simulink model "lane_change_acc_model"  (R2023b)
settings: Solver=ode4  StartTime=0.0  StopTime=T  FixedStep=0.1  RelTol=1e-3
InitFcn:
  | dt = 0.1; T = 20;
  | v_ego0 = 15; d_min = 5; t_headway = 1.2;
  | Kp = 0.5;
  | lane_width = 3.5;
  | mode = 1; % mode = 1 (Keep lane), mode = 2 (Change lane)
  | L = 2.8; K_y = 0.2; K_psi = 1.0;
  | del_actual = 0.2; delta_max = 25*pi/180;
  | 
  | % Lead vehicle and ego car's initial conditions
  | x_lead0 = 30; x_ego0 = 0;
  | v_lead0 = 13;
  | y_lead0 = 0; y_ego0 = 0;
libraries: SignalEditorBlockLib x1
settings Model: Creator=HP  LastModifiedBy=HP

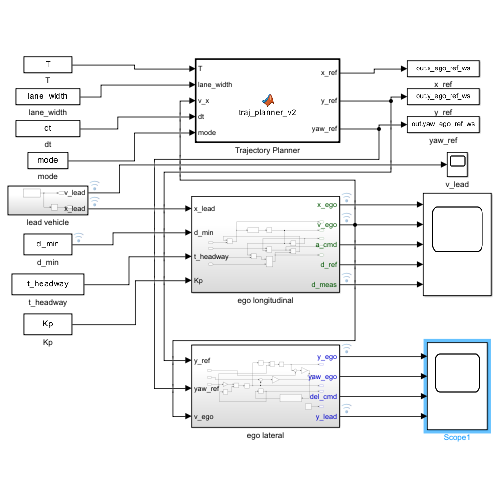
[thumbnail: Simulink's stored preview of the top-level diagram]
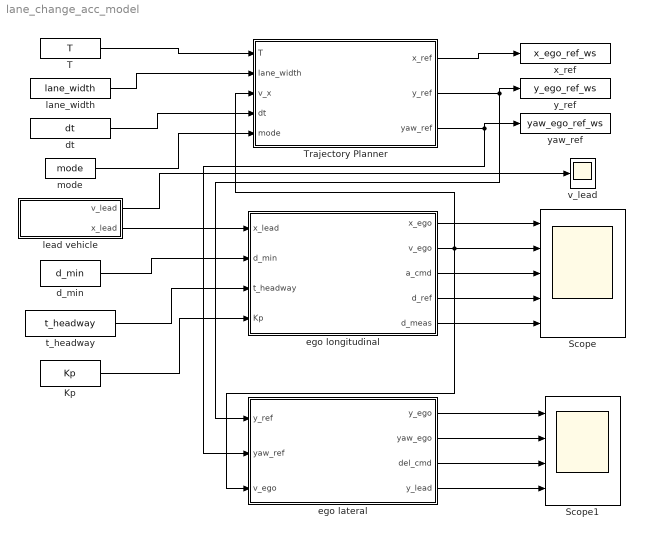
== system lane_change_acc_model ==
  Kp : Constant  Value=Kp
  Scope : Scope  NumInputPorts=5
  Scope1 : Scope  NumInputPorts=4
  T : Constant  Value=T
  Trajectory Planner : MATLAB Function  TreatAsAtomicUnit=on
  d_min : Constant  Value=d_min
  dt : Constant  Value=dt
  ego lateral : Subsystem
  ego longitudinal : Subsystem
  lane_width : Constant  Value=lane_width
  lead vehicle : Subsystem
  mode : Constant  Value=mode
  t_headway : Constant  Value=t_headway
  v_lead : Scope
  x_ref : ToWorkspace  VariableName=x_ego_ref_ws  SaveFormat=Timeseries  SampleTime=-1
  y_ref : ToWorkspace  VariableName=y_ego_ref_ws  SaveFormat=Timeseries  SampleTime=-1
  yaw_ref : ToWorkspace  VariableName=yaw_ego_ref_ws  SaveFormat=Timeseries  SampleTime=-1
  wires:
  Trajectory Planner/2(y_ref) -> y_ref/1, ego lateral/1(y_ref)
  Trajectory Planner/1(x_ref) -> x_ref/1
  T/1 -> Trajectory Planner/1(T)
  lane_width/1 -> Trajectory Planner/2(lane_width)
  dt/1 -> Trajectory Planner/4(dt)
  Trajectory Planner/3(yaw_ref) -> yaw_ref/1, ego lateral/2(yaw_ref)
  d_min/1 -> ego longitudinal/2(d_min)
  t_headway/1 -> ego longitudinal/3(t_headway)
  Kp/1 -> ego longitudinal/4(Kp)
  mode/1 -> Trajectory Planner/5(mode)
  lead vehicle/2(x_lead) -> ego longitudinal/1(x_lead)
  lead vehicle/1(v_lead) -> v_lead/1
  ego longitudinal/2(v_ego) -> ego lateral/3(v_ego), Scope/2, Trajectory Planner/3(v_x)
  ego longitudinal/1(x_ego) -> Scope/1
  ego longitudinal/3(a_cmd) -> Scope/3
  ego longitudinal/5(d_meas) -> Scope/5
  ego lateral/1(y_ego) -> Scope1/1
  ego lateral/2(yaw_ego) -> Scope1/2
  ego lateral/3(del_cmd) -> Scope1/3
  ego longitudinal/4(d_ref) -> Scope/4
  ego lateral/4(y_lead) -> Scope1/4

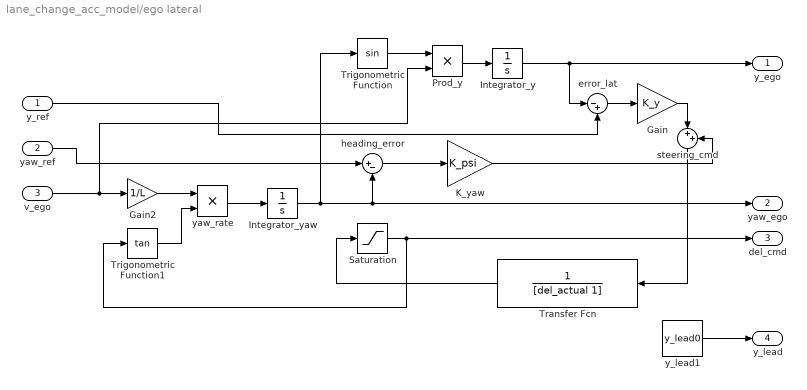
== system lane_change_acc_model/ego lateral ==
  y_ref : Inport
  yaw_ref : Inport  Port=2
  v_ego : Inport  Port=3
  Gain : Gain  Gain=K_y
  Gain2 : Gain  Gain=1/L
  Integrator_y : Integrator
  Integrator_yaw : Integrator
  K_yaw : Gain  Gain=K_psi
  Prod_y : Product
  Saturation : Saturate  UpperLimit=delta_max  LowerLimit=-delta_max
  Transfer Fcn : TransferFcn  Denominator=[del_actual 1]
  Trigonometric Function : Trigonometry
  Trigonometric Function1 : Trigonometry  Operator=tan
  error_lat : Sum  Inputs=|-+
  heading_error : Sum  Inputs=|+-
  steering_cmd : Sum  Inputs=|++
  y_lead1 : Constant  Value=y_lead0
  yaw_rate : Product
  y_ego : Outport
  yaw_ego : Outport  Port=2
  del_cmd : Outport  Port=3
  y_lead : Outport  Port=4
  wires:
  v_ego/1 -> Prod_y/2, Gain2/1
  Gain2/1 -> yaw_rate/1
  Trigonometric Function1/1 -> yaw_rate/2
  yaw_rate/1 -> Integrator_yaw/1
  Integrator_yaw/1 -> heading_error/2, yaw_ego/1, Trigonometric Function/1
  Trigonometric Function/1 -> Prod_y/1
  Prod_y/1 -> Integrator_y/1
  Integrator_y/1 -> error_lat/1, y_ego/1
  y_ref/1 -> error_lat/2
  yaw_ref/1 -> heading_error/1
  error_lat/1 -> Gain/1
  heading_error/1 -> K_yaw/1
  K_yaw/1 -> steering_cmd/2
  Gain/1 -> steering_cmd/1
  steering_cmd/1 -> Transfer Fcn/1
  Transfer Fcn/1 -> Saturation/1
  Saturation/1 -> Trigonometric Function1/1, del_cmd/1
  y_lead1/1 -> y_lead/1

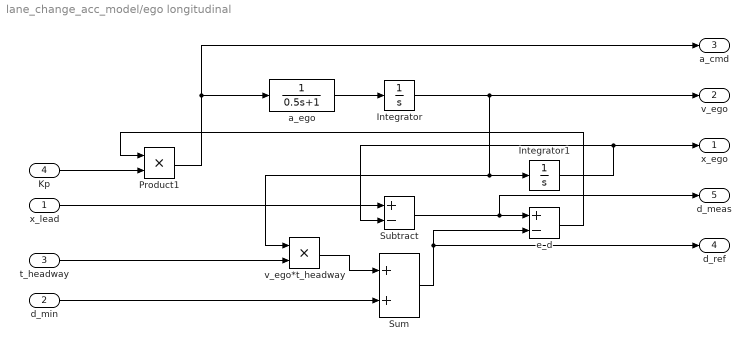
== system lane_change_acc_model/ego longitudinal ==
  x_lead : Inport
  d_min : Inport  Port=2
  t_headway : Inport  Port=3
  Kp : Inport  Port=4
  Integrator : Integrator  InitialCondition=v_ego0
  Integrator1 : Integrator  InitialCondition=x_ego0
  Product1 : Product
  Subtract : Sum  Inputs=+-
  Sum : Sum
  a_ego : TransferFcn  Denominator=[0.5 1]
  e_d : Sum  Inputs=+-
  v_ego*t_headway : Product
  x_ego : Outport
  v_ego : Outport  Port=2
  a_cmd : Outport  Port=3
  d_ref : Outport  Port=4
  d_meas : Outport  Port=5
  wires:
  t_headway/1 -> v_ego*t_headway/2
  v_ego*t_headway/1 -> Sum/1
  d_min/1 -> Sum/2
  x_lead/1 -> Subtract/1
  Subtract/1 -> d_meas/1, e_d/1
  Product1/1 -> a_cmd/1, a_ego/1
  Integrator/1 -> Integrator1/1, v_ego*t_headway/1, v_ego/1
  Sum/1 -> e_d/2, d_ref/1
  a_ego/1 -> Integrator/1
  Integrator1/1 -> Subtract/2, x_ego/1
  e_d/1 -> Product1/1
  Kp/1 -> Product1/2

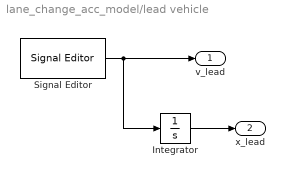
== system lane_change_acc_model/lead vehicle ==
  Integrator : Integrator  InitialCondition=v_lead0
  Signal Editor : SignalEditorBlockLib/Signal Editor  FileName=D:\project\Matlab\cruisecontrol\sim\lead_vehicle_signal.mat  ActiveScenario=Scenario  ActiveSignal=v_lead  IsBus=off  OutputBusObjectStr=Bus: BusObject  SampleTime=0  Interpolate=off  ZeroCross=off  OutputAfterFinalValue=Setting to zero  Unit=inherit  PreserveSignalName=on  ApplySigPropsToAllScenarios=on  ApplySigPropsToAllSignals=off
  v_lead : Outport
  x_lead : Outport  Port=2
  wires:
  Integrator/1 -> x_lead/1
  Signal Editor/1 -> Integrator/1, v_lead/1

== matlab function lane_change_acc_model/Trajectory Planner ==
  settings: updateMethod=DISCRETE
  data: T input; lane_width input; v_x input; dt input; x_ref output; y_ref output; yaw_ref output; mode input
function [x_ref, y_ref, yaw_ref] = traj_planner_v2(T, lane_width, v_x, dt, mode)
% Simulink-safe Trajectory Planner Function
% Generates lane-keeping or lane-change path

%-----------------------------------------------------------
% Persistent declarations
%-----------------------------------------------------------
persistent idx x y yaw N initialized

%-----------------------------------------------------------
% Default initialization (required by Simulink)
%-----------------------------------------------------------
if isempty(idx)
    idx = 1;
end
if isempty(x)
    x = 0;
end
if isempty(y)
    y = 0;
end
if isempty(yaw)
    yaw = 0;
end
if isempty(N)
    N = 1;
end
if isempty(initialized)
    initialized = false;
end

%-----------------------------------------------------------
% Initialize trajectory (runs once per simulation)
%-----------------------------------------------------------
if ~initialized
    % Time vector
    t = 0:dt:T;
    N = numel(t);

    % Longitudinal position
    x = v_x * t;

    % Lateral position based on mode
    if mode == 1
        y = zeros(size(t));          % Keep lane
    else
        y = (lane_width/2) * (1 - cos(pi * t / T));  % Lane change
    end

    % Yaw angle
    dx = [diff(x) 0];
    dy = [diff(y) 0];
    yaw = atan2(dy, dx);

    idx = 1;
    initialized = true;
end

%-----------------------------------------------------------
% Wrap index if exceeds trajectory length
%-----------------------------------------------------------
if idx > N
    idx = 1;
end

%-----------------------------------------------------------
% Output current references
%-----------------------------------------------------------
x_ref = x(idx);
y_ref = y(idx);
yaw_ref = yaw(idx);

%-----------------------------------------------------------
% Increment for next call
%-----------------------------------------------------------
idx = idx + 1;
end
